simulink model "attctrl"  (Simulink 2.20)
settings: Solver=ode45  StartTime=0.0  StopTime=100  MaxStep=.02  RelTol=1e-5  AbsTol=1e-5
values from neighbouring files (symbols this model uses):
  h_off = 0.065    [lvstlage.m]
  h_on = 0.08    [lvstlage.m]
  isat = 480    [lvstlage.m]
  m_stoer = 0.5    [lvstlage.m]
  phi_soll = phi_soll *pi/180    (= 0.0523598775598)    [lvstlage.m]
  TM = 10    [lvstlage.m]
  vr = 10    [lvstlage.m]
libraries: simulink x2
settings Model: SaveTime=off  SaveOutput=off  ConsistencyChecking=off  RTWPlaceOutputsASAP=off

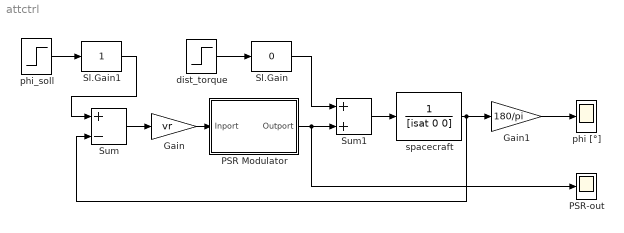
== system attctrl ==
  Gain : Gain  Gain=vr
  Gain1 : Gain  Gain=180/pi
  PSR Modulator : Subsystem
  PSR-out : Scope
      settings: TickLabels=on  TimeRange=auto  YMin=-1.2  YMax=1.2  SaveToWorkspace=off  SaveName=ScopeData  LimitMaxRows=off
  Sl.Gain : simulink/Linear/Slider Gain  low=0  gain=0  high=1
  Sl.Gain1 : simulink/Linear/Slider Gain  low=0  gain=1  high=1
  Sum : Sum  Inputs=+-
  Sum1 : Sum  Inputs=++
  dist_torque : Step  Time=0  Before=0  After=m_stoer
  phi [°] : Scope
      settings: TickLabels=on  TimeRange=auto  YMin=-2  YMax=5  SaveToWorkspace=off  SaveName=ScopeData  LimitMaxRows=off
  phi_soll : Step  Time=0  Before=0  After=phi_soll
  spacecraft : TransferFcn  Numerator=[1]  Denominator=[isat 0 0]
  wires:
  Gain1/1 -> phi [°]/1
  Sum1/1 -> spacecraft/1
  Sum/1 -> Gain/1
  spacecraft/1 -> Gain1/1, Sum/2
  dist_torque/1 -> Sl.Gain/1
  Sl.Gain/1 -> Sum1/1
  phi_soll/1 -> Sl.Gain1/1
  Sl.Gain1/1 -> Sum/1
  Gain/1 -> PSR Modulator/1(Inport)
  PSR Modulator/1(Outport) -> Sum1/2, PSR-out/1

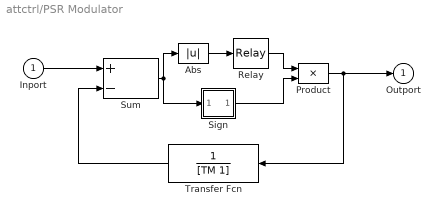
== system attctrl/PSR Modulator ==
  Inport : Inport  Port=1  PortWidth=-1  SampleTime=-1
  Abs : Abs
  Product : Product  Inputs=2
  Relay : Relay  OnSwitchValue=h_on  OffSwitchValue=h_off  OnOutputValue=b  OffOutputValue=0
  Sign : Subsystem
      mask Type: Sign
      mask Description: y = sign(x)
      mask Help: Sign Function:\n\t\t\ty = 1 if x > 0\n\t\t\ty = 0 if x = 0\n\t\t\ty = -1 if x < 0
      mask Display: plot(-50,-50,50,50,[-50,50],[0,0],[0,0],[-50,50],[-40,0],[-30,-30],[0,40],[30,30])
  Sum : Sum  Inputs=+-
  Transfer Fcn : TransferFcn  Orientation=left  Numerator=[1]  Denominator=[TM 1]
  Outport : Outport  Port=1  InitialOutput=0
  wires:
  Abs/1 -> Relay/1
  Relay/1 -> Product/1
  Inport/1 -> Sum/1
  Sign/1(out_1) -> Product/2
  Transfer Fcn/1 -> Sum/2
  Product/1 -> Outport/1, Transfer Fcn/1
  Sum/1 -> Abs/1, Sign/1(in_1)

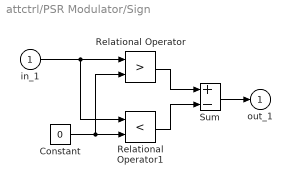
== system attctrl/PSR Modulator/Sign ==
  in_1 : Inport  Port=1  PortWidth=-1  SampleTime=-1
  Constant : Constant  Value=0
  Relational Operator : RelationalOperator  Operator=>
  Relational Operator1 : RelationalOperator  Operator=<
  Sum : Sum  Inputs=+-
  out_1 : Outport  Port=1  InitialOutput=0
  wires:
  in_1/1 -> Relational Operator/1, Relational Operator1/1
  Constant/1 -> Relational Operator1/2, Relational Operator/2
  Relational Operator1/1 -> Sum/2
  Relational Operator/1 -> Sum/1
  Sum/1 -> out_1/1
